simulink model "SF050A_MotTqTranlDampg"  (R2013b)
settings: Solver=FixedStepDiscrete  SolverMode=SingleTasking  StartTime=0.0  StopTime=29  FixedStep=.002  RelTol=1e-3
undefined symbols (not defined in the file): LoaSt1, MotTqTranlDampgCmdLim, MotTqTranlDampgDampgCoeff, MotTqTranlDampgRampEnd, MotTqTranlDampgTmrPt1, MotTqTranlDampgTmrPt2, MotTqTranlDampgVelThd, RAMPSTRT_ULS_U2P14, SYSGLBPRM_MOTTQCMDHILIM_MOTNWTMTR_F32, SYSGLBPRM_MOTTQCMDLOLIM_MOTNWTMTR_F32, SysSt1, TICNVN_MILLISECPERCNT_F32
libraries: simulink x8, FloatToFixd x4, FixdToFloat x3, NxtrSign x2, NxtrAbslt x1, LnrIntrpnDyn x1, LnrIntrpn x1
Description:
  | This FDD describes the controlled disable damping shutdown method used in the
  | EPS system for torque sensor failures.  When the torque sensor fails, an output
  | torque is computed based on motor velocity to reduce the amount of “handwheel
  | kick” perceived by the driver.
settings Model: Creator=Kevin Derry  LastModifiedBy=XZB1DB
settings OptimizationCC: ExpressionDepthLimit=2147483647

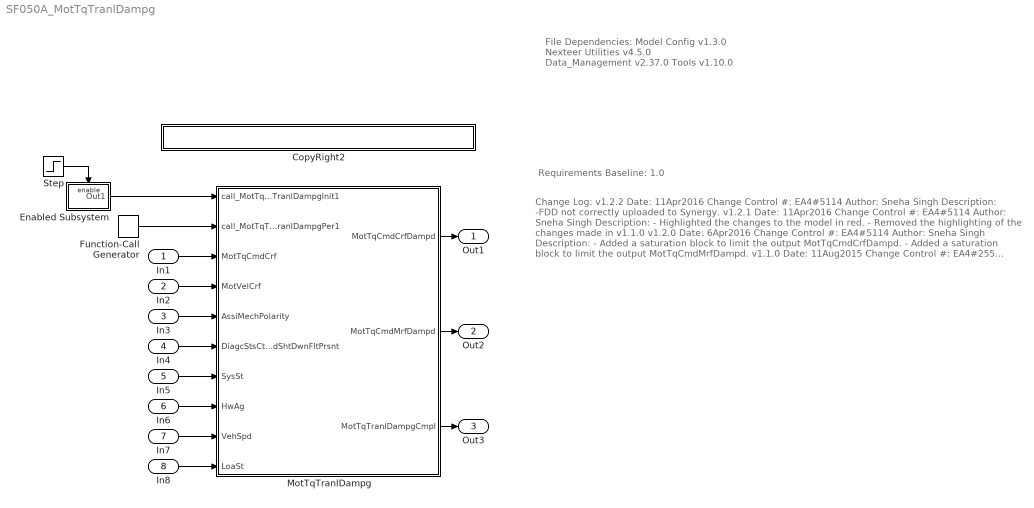
== system SF050A_MotTqTranlDampg ==
  note: File Dependencies:
      |
      | Model Config v1.3.0
      | Nexteer Utilities v4.5.0
      | Data_Management v2.37.0
      | Tools v1.10.0
  note: Requirements Baseline: 1.0
  note: Change Log:
      |
      | v1.2.2
      | Date: 11Apr2016
      | Change Control #: EA4#5114
      | Author: Sneha Singh
      | Description:
      | -FDD not correctly uploaded to Synergy.
      |
      | v1.2.1
      | Date: 11Apr2016
      | Change Control #: EA4#5114
      | Author: Sneha Singh
      | Description:
      | - Highlighted the changes to the model in red.
      | - Removed the highlighting of the changes made in v1.1.0
      |
      | v1.2.0
      | Date: 6Apr2016
      | Change Control #: EA4#5114
      | Author: Sneha Singh
      | Description:
      | - Added a saturation block to limit the output MotTqCmdCrfDampd.
      | - Added a saturation block to limit the output MotTqCmdMrfDampd.
      |
      | v1.1.0
      | Date:  11Aug2015
      | Change Control #: EA4#255
      | Author:  Kevin Derry
      | Description:
      | -  Datatype of CtrldDampgScaY was u16p0, now u2p14.
      | -  New RAMPSTRT constant used instead of hardcoded "1".
      | -  FixdToFloat after CtrldDampgSca interpolation was u16p0, now u2p14.
      | -  Verbiage of Reset Timer block reworded for clarity.
      | -  SwOutputCntrl block rearranged for clarity.  No functional change.
      | -  Datatype of cal MotTqTranlDampgRampEnd was f32, now u2p14.
      | -  Removed two FloatToFixd in MotTqTranlDampgInit1 runnable.
      |
      | v1.0.0
      | Date: 18July2015
      | Change Control #: EA4#255
      | Author:  Kevin Derry
      | Description:
      | - Initial Release, based on EA3 v002
      | - This is a "level zero" model, not fully compliant with
      |   EA4 standards (or even close to it, for that matter).
  In1 : Inport
  In2 : Inport  Port=2
  In3 : Inport  Port=3
  In4 : Inport  Port=4
  In5 : Inport  Port=5  OutDataTypeStr=Enum: SysSt1
  In6 : Inport  Port=6
  In7 : Inport  Port=7
  In8 : Inport  Port=8
  CopyRight2 : Subsystem  Description=|  mask(Copyright Information){none=on}
      | Copyright info block.                                               
      |                                                                     
      | Place copyright information at the top of every subsystem in design.
      mask prompts: none "No parameters"
      mask help: Place copyright information at the top of every subsystem in design.
      mask Display:
      | NxtrConf = 'Nexteer Confidential';
      | 
      | sys = bdroot; %handle for the current model ("system")
      | first = get_param(sys,'Created');
      | if(isempty(first))
      |     first = datestr(now,'yyyy');
      | else
      |     first = first(end-3:end);  %year is last four digits
      | end
      | 
      | last = get_param(sys,'LastModifiedDate');
      | if isempty(last)
      |     last = datestr(now,'yyyy');
      | else
      |     last = last(end-3:end);
      | end
      | 
      | if strcmp(first,last)
      |     fprintf('%s -- Copyright %s Nexteer',NxtrConf,first)
      | else
      |     fprintf('%s -- %s%s- %s Nexteer',NxtrConf,char(169),first,last)
      | end
  Enabled Subsystem : Subsystem  TreatAsAtomicUnit=on
  Function-Call Generator : simulink/Ports & Subsystems/Function-Call Generator  sample_time=.002  numberOfIterations=1
  MotTqTranlDampg : Subsystem
  Step : Step  Time=.0000001  Before=1  After=0  SampleTime=0
  Out1 : Outport
  Out2 : Outport  Port=2
  Out3 : Outport  Port=3
  wires:
  In8/1 -> MotTqTranlDampg/10(LoaSt)
  MotTqTranlDampg/1(MotTqCmdCrfDampd) -> Out1/1
  In5/1 -> MotTqTranlDampg/7(SysSt)
  In4/1 -> MotTqTranlDampg/6(DiagcStsCtrldShtDwnFltPrsnt)
  In6/1 -> MotTqTranlDampg/8(HwAg)
  In3/1 -> MotTqTranlDampg/5(AssiMechPolarity)
  In7/1 -> MotTqTranlDampg/9(VehSpd)
  In2/1 -> MotTqTranlDampg/4(MotVelCrf)
  In1/1 -> MotTqTranlDampg/3(MotTqCmdCrf)
  MotTqTranlDampg/2(MotTqCmdMrfDampd) -> Out2/1
  MotTqTranlDampg/3(MotTqTranlDampgCmpl) -> Out3/1
  Function-Call Generator/1 -> MotTqTranlDampg/2(call_MotTqTranlDampgPer1)
  Step/1 -> Enabled Subsystem/Enable
  Enabled Subsystem/1(Out1) -> MotTqTranlDampg/1(call_MotTqTranlDampgInit1)

== system SF050A_MotTqTranlDampg/CopyRight2 ==

== system SF050A_MotTqTranlDampg/Enabled Subsystem ==
  Enable : EnablePort
  Function-Call Generator1 : simulink/Ports & Subsystems/Function-Call Generator  sample_time=.002  numberOfIterations=1
  Out1 : Outport
  wires:
  Function-Call Generator1/1 -> Out1/1

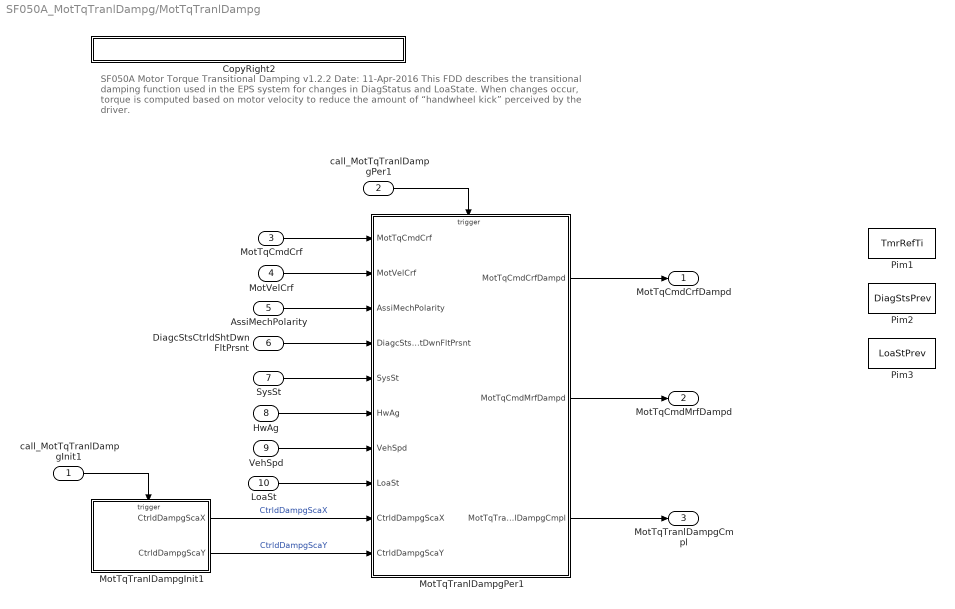
== system SF050A_MotTqTranlDampg/MotTqTranlDampg ==
  note: SF050A  Motor Torque Transitional Damping
      | v1.2.2      Date: 11-Apr-2016
      |
      | This FDD describes the transitional damping function used in the EPS system for changes in DiagStatus and LoaState.  When changes occur,
      | torque is computed based on motor velocity to reduce the amount of “handwheel kick” perceived by the driver.
  call_MotTqTranlDampgInit1 : Inport
  call_MotTqTranlDampgPer1 : Inport  Port=2
  MotTqCmdCrf : Inport  Port=3
  MotVelCrf : Inport  Port=4
  AssiMechPolarity : Inport  Port=5
  DiagcStsCtrldShtDwnFltPrsnt : Inport  Port=6
  SysSt : Inport  Port=7
  HwAg : Inport  Port=8
  VehSpd : Inport  Port=9
  LoaSt : Inport  Port=10
  CopyRight2 : Subsystem  Description=|  mask(Copyright Information){none=on}
      | Copyright info block.                                               
      |                                                                     
      | Place copyright information at the top of every subsystem in design.
      mask prompts: none "No parameters"
      mask help: Place copyright information at the top of every subsystem in design.
      mask Display:
      | NxtrConf = 'Nexteer Confidential';
      | 
      | sys = bdroot; %handle for the current model ("system")
      | first = get_param(sys,'Created');
      | if(isempty(first))
      |     first = datestr(now,'yyyy');
      | else
      |     first = first(end-3:end);  %year is last four digits
      | end
      | 
      | last = get_param(sys,'LastModifiedDate');
      | if isempty(last)
      |     last = datestr(now,'yyyy');
      | else
      |     last = last(end-3:end);
      | end
      | 
      | if strcmp(first,last)
      |     fprintf('%s -- Copyright %s Nexteer',NxtrConf,first)
      | else
      |     fprintf('%s -- %s%s- %s Nexteer',NxtrConf,char(169),first,last)
      | end
  MotTqTranlDampgInit1 : Subsystem
  MotTqTranlDampgPer1 : Subsystem
  Pim1 : DataStoreMemory  DataStoreName=TmrRefTi  ReadBeforeWriteMsg=warning  WriteAfterWriteMsg=warning  WriteAfterReadMsg=warning  StateMustResolveToSignalObject=on
  Pim2 : DataStoreMemory  DataStoreName=DiagStsPrev  ReadBeforeWriteMsg=warning  WriteAfterWriteMsg=warning  WriteAfterReadMsg=warning  StateMustResolveToSignalObject=on
  Pim3 : DataStoreMemory  DataStoreName=LoaStPrev  ReadBeforeWriteMsg=warning  WriteAfterWriteMsg=warning  WriteAfterReadMsg=warning  InitialValue=LoaSt1.LOAST_NORM  OutDataTypeStr=Enum: LoaSt1  StateMustResolveToSignalObject=on
  MotTqCmdCrfDampd : Outport
  MotTqCmdMrfDampd : Outport  Port=2
  MotTqTranlDampgCmpl : Outport  Port=3
  wires:
  MotTqCmdCrf/1 -> MotTqTranlDampgPer1/1(MotTqCmdCrf)
  MotVelCrf/1 -> MotTqTranlDampgPer1/2(MotVelCrf)
  AssiMechPolarity/1 -> MotTqTranlDampgPer1/3(AssiMechPolarity)
  DiagcStsCtrldShtDwnFltPrsnt/1 -> MotTqTranlDampgPer1/4(DiagcStsCtrldShtDwnFltPrsnt)
  SysSt/1 -> MotTqTranlDampgPer1/5(SysSt)
  HwAg/1 -> MotTqTranlDampgPer1/6(HwAg)
  VehSpd/1 -> MotTqTranlDampgPer1/7(VehSpd)
  LoaSt/1 -> MotTqTranlDampgPer1/8(LoaSt)
  MotTqTranlDampgPer1/1(MotTqCmdCrfDampd) -> MotTqCmdCrfDampd/1
  MotTqTranlDampgPer1/2(MotTqCmdMrfDampd) -> MotTqCmdMrfDampd/1
  MotTqTranlDampgPer1/3(MotTqTranlDampgCmpl) -> MotTqTranlDampgCmpl/1
  MotTqTranlDampgInit1/1(CtrldDampgScaX) -> MotTqTranlDampgPer1/9(CtrldDampgScaX)  "CtrldDampgScaX"
  MotTqTranlDampgInit1/2(CtrldDampgScaY) -> MotTqTranlDampgPer1/10(CtrldDampgScaY)  "CtrldDampgScaY"
  call_MotTqTranlDampgInit1/1 -> MotTqTranlDampgInit1/Trigger
  call_MotTqTranlDampgPer1/1 -> MotTqTranlDampgPer1/Trigger

== system SF050A_MotTqTranlDampg/MotTqTranlDampg/CopyRight2 ==

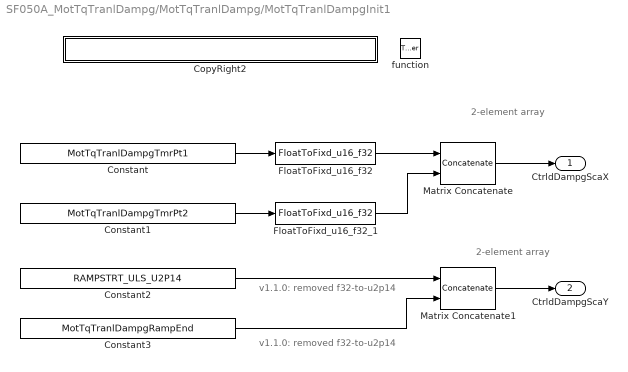
== system SF050A_MotTqTranlDampg/MotTqTranlDampg/MotTqTranlDampgInit1 ==
  note: v1.1.0: removed f32-to-u2p14
  note: 2-element array
  note: 2-element array
  note: v1.1.0: removed f32-to-u2p14
  function : TriggerPort  TriggerType=function-call
  Constant : Constant  Value=MotTqTranlDampgTmrPt1
  Constant1 : Constant  Value=MotTqTranlDampgTmrPt2
  Constant2 : Constant  Value=RAMPSTRT_ULS_U2P14
  Constant3 : Constant  Value=MotTqTranlDampgRampEnd
  CopyRight2 : Subsystem  Description=|  mask(Copyright Information){none=on}
      | Copyright info block.                                               
      |                                                                     
      | Place copyright information at the top of every subsystem in design.
      mask prompts: none "No parameters"
      mask help: Place copyright information at the top of every subsystem in design.
      mask Display:
      | NxtrConf = 'Nexteer Confidential';
      | 
      | sys = bdroot; %handle for the current model ("system")
      | first = get_param(sys,'Created');
      | if(isempty(first))
      |     first = datestr(now,'yyyy');
      | else
      |     first = first(end-3:end);  %year is last four digits
      | end
      | 
      | last = get_param(sys,'LastModifiedDate');
      | if isempty(last)
      |     last = datestr(now,'yyyy');
      | else
      |     last = last(end-3:end);
      | end
      | 
      | if strcmp(first,last)
      |     fprintf('%s -- Copyright %s Nexteer',NxtrConf,first)
      | else
      |     fprintf('%s -- %s%s- %s Nexteer',NxtrConf,char(169),first,last)
      | end
  FloatToFixd_u16_f32 : FloatToFixd/FloatToFixd_u16_f32  Param1=0
  FloatToFixd_u16_f32_1 : FloatToFixd/FloatToFixd_u16_f32  Param1=0
  Matrix Concatenate : Concatenate
  Matrix Concatenate1 : Concatenate
  CtrldDampgScaX : Outport
  CtrldDampgScaY : Outport  Port=2
  wires:
  Constant/1 -> FloatToFixd_u16_f32/1
  Constant1/1 -> FloatToFixd_u16_f32_1/1
  FloatToFixd_u16_f32/1 -> Matrix Concatenate/1
  FloatToFixd_u16_f32_1/1 -> Matrix Concatenate/2
  Constant2/1 -> Matrix Concatenate1/1
  Constant3/1 -> Matrix Concatenate1/2
  Matrix Concatenate1/1 -> CtrldDampgScaY/1
  Matrix Concatenate/1 -> CtrldDampgScaX/1

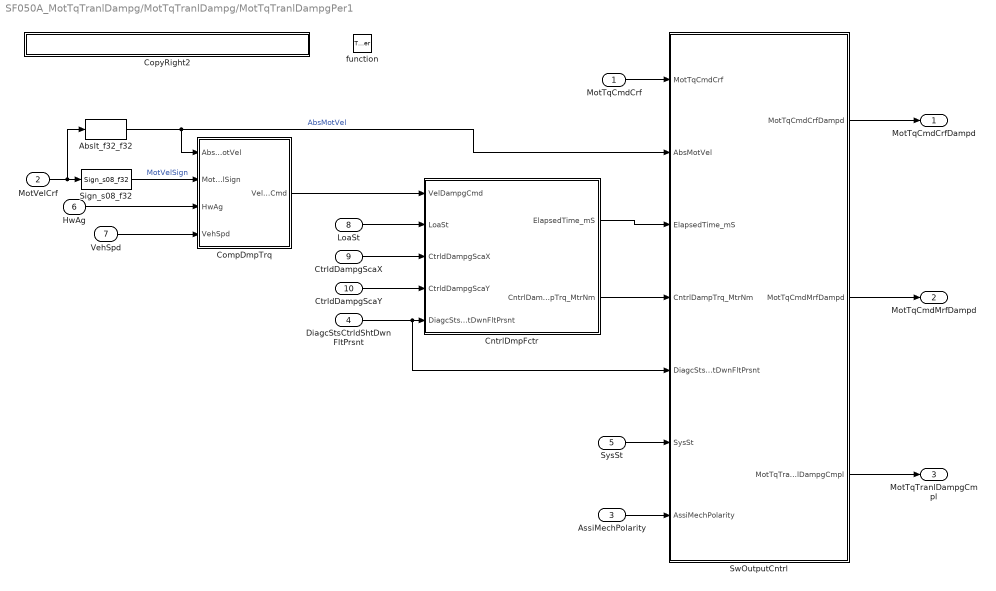
== system SF050A_MotTqTranlDampg/MotTqTranlDampg/MotTqTranlDampgPer1 ==
  MotTqCmdCrf : Inport
  MotVelCrf : Inport  Port=2
  AssiMechPolarity : Inport  Port=3
  DiagcStsCtrldShtDwnFltPrsnt : Inport  Port=4
  SysSt : Inport  Port=5
  HwAg : Inport  Port=6
  VehSpd : Inport  Port=7
  LoaSt : Inport  Port=8
  CtrldDampgScaX : Inport  Port=9
  CtrldDampgScaY : Inport  Port=10
  function : TriggerPort  TriggerType=function-call
  Abslt_f32_f32 : NxtrAbslt/Abslt_f32_f32  SFunctionSpec=single y1 = Abslt_f32_f32(single u1)
      settings: AttributesFormatString=%<Name>
  CntrlDmpFctr : Subsystem  Tag=Control Damping Factor
      settings: AttributesFormatString=%<Tag>
  CompDmpTrq : Subsystem  Tag=Compute Damping Torque
      settings: AttributesFormatString=%<Tag>
  CopyRight2 : Subsystem  Description=|  mask(Copyright Information){none=on}
      | Copyright info block.                                               
      |                                                                     
      | Place copyright information at the top of every subsystem in design.
      mask prompts: none "No parameters"
      mask help: Place copyright information at the top of every subsystem in design.
      mask Display:
      | NxtrConf = 'Nexteer Confidential';
      | 
      | sys = bdroot; %handle for the current model ("system")
      | first = get_param(sys,'Created');
      | if(isempty(first))
      |     first = datestr(now,'yyyy');
      | else
      |     first = first(end-3:end);  %year is last four digits
      | end
      | 
      | last = get_param(sys,'LastModifiedDate');
      | if isempty(last)
      |     last = datestr(now,'yyyy');
      | else
      |     last = last(end-3:end);
      | end
      | 
      | if strcmp(first,last)
      |     fprintf('%s -- Copyright %s Nexteer',NxtrConf,first)
      | else
      |     fprintf('%s -- %s%s- %s Nexteer',NxtrConf,char(169),first,last)
      | end
  Sign_s08_f32 : NxtrSign/Sign_s08_f32  SFunctionSpec=int8 y1 = Sign_s08_f32(single u1)
  SwOutputCntrl : Subsystem  Tag=Switch Output Control
      settings: AttributesFormatString=%<Tag>
  MotTqCmdCrfDampd : Outport
  MotTqCmdMrfDampd : Outport  Port=2
  MotTqTranlDampgCmpl : Outport  Port=3
  wires:
  DiagcStsCtrldShtDwnFltPrsnt/1 -> SwOutputCntrl/5(DiagcStsCtrldShtDwnFltPrsnt), CntrlDmpFctr/5(DiagcStsCtrldShtDwnFltPrsnt)
  LoaSt/1 -> CntrlDmpFctr/2(LoaSt)
  SysSt/1 -> SwOutputCntrl/6(SysSt)
  CntrlDmpFctr/2(CntrlDampTrq_MtrNm) -> SwOutputCntrl/4(CntrlDampTrq_MtrNm)
  CompDmpTrq/1(VelDampgCmd) -> CntrlDmpFctr/1(VelDampgCmd)
  MotTqCmdCrf/1 -> SwOutputCntrl/1(MotTqCmdCrf)
  SwOutputCntrl/1(MotTqCmdCrfDampd) -> MotTqCmdCrfDampd/1
  SwOutputCntrl/2(MotTqCmdMrfDampd) -> MotTqCmdMrfDampd/1
  SwOutputCntrl/3(MotTqTranlDampgCmpl) -> MotTqTranlDampgCmpl/1
  CntrlDmpFctr/1(ElapsedTime_mS) -> SwOutputCntrl/3(ElapsedTime_mS)
  AssiMechPolarity/1 -> SwOutputCntrl/7(AssiMechPolarity)
  CtrldDampgScaX/1 -> CntrlDmpFctr/3(CtrldDampgScaX)
  CtrldDampgScaY/1 -> CntrlDmpFctr/4(CtrldDampgScaY)
  MotVelCrf/1 -> Abslt_f32_f32/1, Sign_s08_f32/1
  Sign_s08_f32/1 -> CompDmpTrq/2(MotVelSign)  "MotVelSign"
  Abslt_f32_f32/1 -> CompDmpTrq/1(AbsMotVel), SwOutputCntrl/2(AbsMotVel)  "AbsMotVel"
  HwAg/1 -> CompDmpTrq/3(HwAg)
  VehSpd/1 -> CompDmpTrq/4(VehSpd)

== system SF050A_MotTqTranlDampg/MotTqTranlDampg/MotTqTranlDampgInit1/CopyRight2 ==

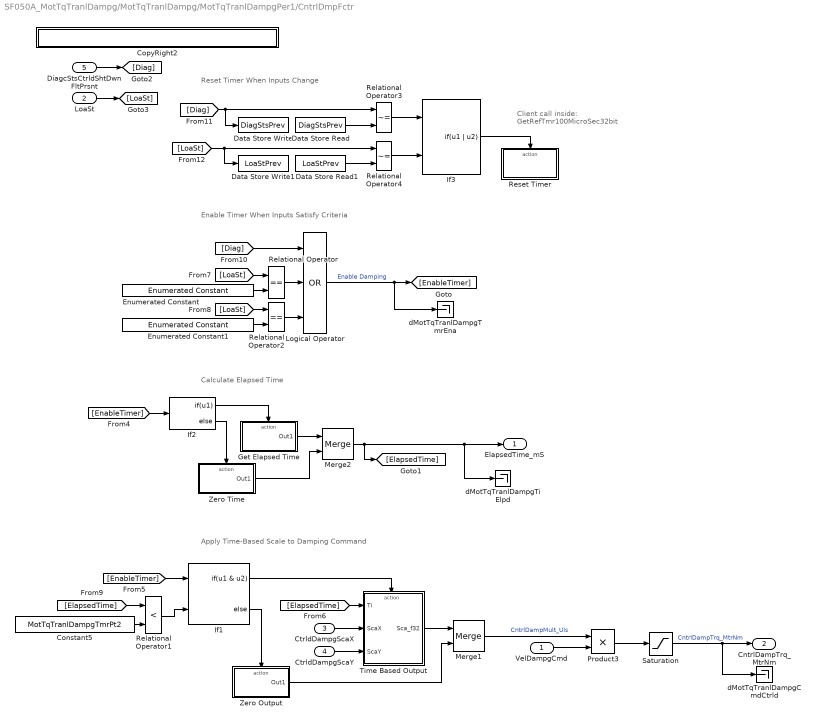
== system SF050A_MotTqTranlDampg/MotTqTranlDampg/MotTqTranlDampgPer1/CntrlDmpFctr ==
  note: Reset Timer When Inputs Change
  note: Client call inside:
      | GetRefTmr100MicroSec32bit
  note: Enable Timer When Inputs Satisfy Criteria
  note: Calculate Elapsed Time
  note: Apply Time-Based Scale to Damping Command
  VelDampgCmd : Inport
  LoaSt : Inport  Port=2
  CtrldDampgScaX : Inport  Port=3
  CtrldDampgScaY : Inport  Port=4
  DiagcStsCtrldShtDwnFltPrsnt : Inport  Port=5
  Constant5 : Constant  Value=MotTqTranlDampgTmrPt2
  CopyRight2 : Subsystem  Description=|  mask(Copyright Information){none=on}
      | Copyright info block.                                               
      |                                                                     
      | Place copyright information at the top of every subsystem in design.
      mask prompts: none "No parameters"
      mask help: Place copyright information at the top of every subsystem in design.
      mask Display:
      | NxtrConf = 'Nexteer Confidential';
      | 
      | sys = bdroot; %handle for the current model ("system")
      | first = get_param(sys,'Created');
      | if(isempty(first))
      |     first = datestr(now,'yyyy');
      | else
      |     first = first(end-3:end);  %year is last four digits
      | end
      | 
      | last = get_param(sys,'LastModifiedDate');
      | if isempty(last)
      |     last = datestr(now,'yyyy');
      | else
      |     last = last(end-3:end);
      | end
      | 
      | if strcmp(first,last)
      |     fprintf('%s -- Copyright %s Nexteer',NxtrConf,first)
      | else
      |     fprintf('%s -- %s%s- %s Nexteer',NxtrConf,char(169),first,last)
      | end
  Data Store Read : DataStoreRead  Priority=1  DataStoreName=DiagStsPrev
  Data Store Read1 : DataStoreRead  Priority=1  DataStoreName=LoaStPrev
  Data Store Write : DataStoreWrite  Priority=2  DataStoreName=DiagStsPrev
  Data Store Write1 : DataStoreWrite  Priority=2  DataStoreName=LoaStPrev
  Enumerated Constant : simulink/Sources/Enumerated Constant  OutDataTypeStr=Enum: LoaSt1  Value=LoaSt1.LOAST_SWBASDMTGTN  SampleTime=inf
  Enumerated Constant1 : simulink/Sources/Enumerated Constant  OutDataTypeStr=Enum: LoaSt1  Value=LoaSt1.LOAST_FADEOUT  SampleTime=inf
  Get Elapsed Time : Subsystem  TreatAsAtomicUnit=on
  If1 : If  NumInputs=2  IfExpression=u1 & u2
  If2 : If  IfExpression=u1
  If3 : If  NumInputs=2  IfExpression=u1 | u2  ShowElse=off
  Logical Operator : Logic  Operator=OR  Inputs=3  AllPortsSameDT=off  OutDataTypeStr=boolean
  Merge1 : Merge
  Merge2 : Merge
  Product3 : Product  RndMeth=Zero
  Relational Operator : RelationalOperator  Operator===  OutDataTypeStr=boolean
  Relational Operator1 : RelationalOperator  Operator=<  OutDataTypeStr=boolean
  Relational Operator2 : RelationalOperator  Operator===  OutDataTypeStr=boolean
  Relational Operator3 : RelationalOperator  Operator=~=  OutDataTypeStr=boolean
  Relational Operator4 : RelationalOperator  Operator=~=  OutDataTypeStr=boolean
  Reset Timer : Subsystem  TreatAsAtomicUnit=on
  Saturation : Saturate  UpperLimit=MotTqTranlDampgCmdLim  LowerLimit=-MotTqTranlDampgCmdLim
      settings: AttributesFormatString=%<UpperLimit>\n%<LowerLimit>
  Time Based Output : Subsystem  TreatAsAtomicUnit=on
  Zero Output : Subsystem  TreatAsAtomicUnit=on
  Zero Time : Subsystem  TreatAsAtomicUnit=on
  dMotTqTranlDampgCmdCtrld : Terminator
  "dMotTqTranlDampgTiElpd   " : Terminator
  "dMotTqTranlDampgTmrEna   " : Terminator
  ElapsedTime_mS : Outport
  CntrlDampTrq_MtrNm : Outport  Port=2
  wires:
  Saturation/1 -> dMotTqTranlDampgCmdCtrld/1, CntrlDampTrq_MtrNm/1  "CntrlDampTrq_MtrNm"
  Constant5/1 -> Relational Operator1/2
  Merge1/1 -> Product3/1  "CntrlDampMult_Uls"
  VelDampgCmd/1 -> Product3/2
  Product3/1 -> Saturation/1
  DiagcStsCtrldShtDwnFltPrsnt/1 -> [Diag]
  Merge2/1 -> ElapsedTime_mS/1, "dMotTqTranlDampgTiElpd   "/1, [ElapsedTime]
  [ElapsedTime] -> Relational Operator1/1
  Relational Operator1/1 -> If1/2
  Enumerated Constant/1 -> Relational Operator/2
  Enumerated Constant1/1 -> Relational Operator2/2
  [ElapsedTime] -> Time Based Output/1(Ti)
  CtrldDampgScaX/1 -> Time Based Output/2(ScaX)
  CtrldDampgScaY/1 -> Time Based Output/3(ScaY)
  If1/1 -> Time Based Output/Action
  [EnableTimer] -> If1/1
  If1/2 -> Zero Output/Action
  Time Based Output/1(Sca_f32) -> Merge1/1
  Zero Output/1(Out1) -> Merge1/2
  [EnableTimer] -> If2/1
  If2/2 -> Zero Time/Action
  If2/1 -> Get Elapsed Time/Action
  Get Elapsed Time/1(Out1) -> Merge2/1
  Zero Time/1(Out1) -> Merge2/2
  Logical Operator/1 -> [EnableTimer], "dMotTqTranlDampgTmrEna   "/1  "Enable Damping"
  LoaSt/1 -> [LoaSt]
  [LoaSt] -> Relational Operator/1
  [LoaSt] -> Relational Operator2/1
  Relational Operator/1 -> Logical Operator/2
  Relational Operator2/1 -> Logical Operator/3
  [Diag] -> Logical Operator/1
  [Diag] -> Data Store Write/1, Relational Operator3/1
  Data Store Read1/1 -> Relational Operator4/2
  [LoaSt] -> Data Store Write1/1, Relational Operator4/1
  Relational Operator3/1 -> If3/1
  Relational Operator4/1 -> If3/2
  If3/1 -> Reset Timer/Action
  Data Store Read/1 -> Relational Operator3/2

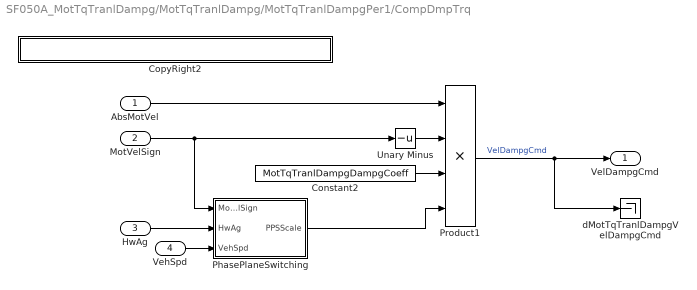
== system SF050A_MotTqTranlDampg/MotTqTranlDampg/MotTqTranlDampgPer1/CompDmpTrq ==
  AbsMotVel : Inport
  MotVelSign : Inport  Port=2
  HwAg : Inport  Port=3
  VehSpd : Inport  Port=4
  Constant2 : Constant  Value=MotTqTranlDampgDampgCoeff
  CopyRight2 : Subsystem  Description=|  mask(Copyright Information){none=on}
      | Copyright info block.                                               
      |                                                                     
      | Place copyright information at the top of every subsystem in design.
      mask prompts: none "No parameters"
      mask help: Place copyright information at the top of every subsystem in design.
      mask Display:
      | NxtrConf = 'Nexteer Confidential';
      | 
      | sys = bdroot; %handle for the current model ("system")
      | first = get_param(sys,'Created');
      | if(isempty(first))
      |     first = datestr(now,'yyyy');
      | else
      |     first = first(end-3:end);  %year is last four digits
      | end
      | 
      | last = get_param(sys,'LastModifiedDate');
      | if isempty(last)
      |     last = datestr(now,'yyyy');
      | else
      |     last = last(end-3:end);
      | end
      | 
      | if strcmp(first,last)
      |     fprintf('%s -- Copyright %s Nexteer',NxtrConf,first)
      | else
      |     fprintf('%s -- %s%s- %s Nexteer',NxtrConf,char(169),first,last)
      | end
  PhasePlaneSwitching : Subsystem
  Product1 : Product  Inputs=4  OutDataTypeStr=single  RndMeth=Zero
  Unary Minus : UnaryMinus
  "dMotTqTranlDampgVelDampgCmd " : Terminator
  VelDampgCmd : Outport
  wires:
  MotVelSign/1 -> Unary Minus/1, PhasePlaneSwitching/1(MotVelSign)
  Unary Minus/1 -> Product1/2
  Product1/1 -> "dMotTqTranlDampgVelDampgCmd "/1, VelDampgCmd/1  "VelDampgCmd"
  Constant2/1 -> Product1/3
  HwAg/1 -> PhasePlaneSwitching/2(HwAg)
  VehSpd/1 -> PhasePlaneSwitching/3(VehSpd)
  PhasePlaneSwitching/1(PPSScale) -> Product1/4
  AbsMotVel/1 -> Product1/1

== system SF050A_MotTqTranlDampg/MotTqTranlDampg/MotTqTranlDampgPer1/CopyRight2 ==

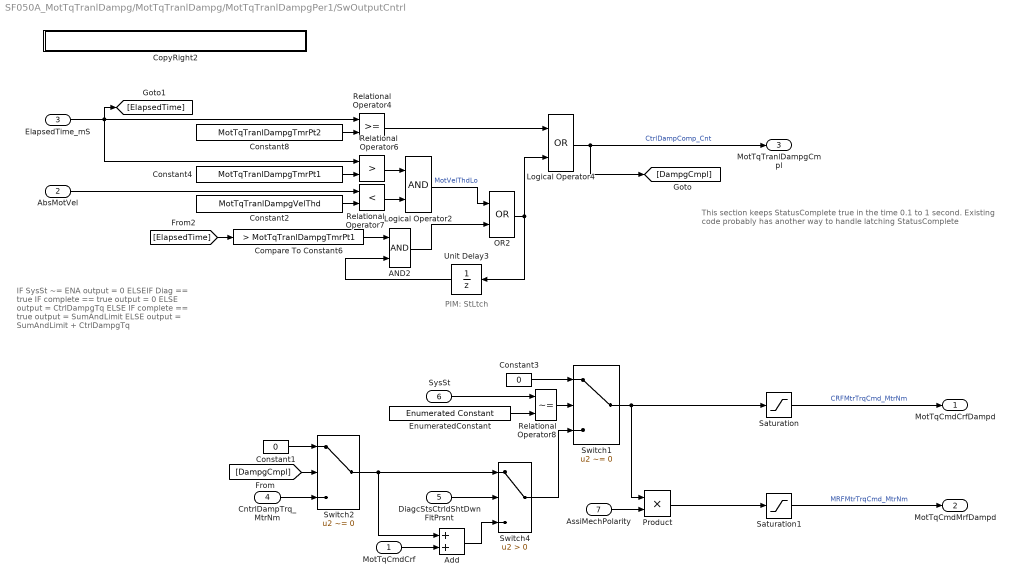
== system SF050A_MotTqTranlDampg/MotTqTranlDampg/MotTqTranlDampgPer1/SwOutputCntrl ==
  note: PIM: StLtch
  note: IF  SysSt ~= ENA
      |    output = 0
      | ELSEIF  Diag == true
      |    IF  complete == true
      |        output = 0
      |    ELSE
      |        output = CtrlDampgTq
      | ELSE
      |    IF  complete == true
      |        output = SumAndLimit
      |    ELSE
      |        output = SumAndLimit + CtrlDampgTq
  note: This section keeps StatusComplete true in the time 0.1 to 1 second.
      | Existing code probably has another way to handle latching StatusComplete
  MotTqCmdCrf : Inport
  AbsMotVel : Inport  Port=2
  ElapsedTime_mS : Inport  Port=3
  CntrlDampTrq_MtrNm : Inport  Port=4
  DiagcStsCtrldShtDwnFltPrsnt : Inport  Port=5
  SysSt : Inport  Port=6
  AssiMechPolarity : Inport  Port=7
  AND2 : Logic  AllPortsSameDT=off
  Add : Sum
  Compare To Constant6 : simulink/Logic and Bit Operations/Compare To Constant  relop=>  const=MotTqTranlDampgTmrPt1  OutDataTypeStr=boolean
  Constant1 : Constant  Value=0  OutDataTypeStr=single
  Constant2 : Constant  Value=MotTqTranlDampgVelThd
  Constant3 : Constant  Value=0  OutDataTypeStr=single
  Constant4 : Constant  Value=MotTqTranlDampgTmrPt1
  Constant8 : Constant  Value=MotTqTranlDampgTmrPt2
  CopyRight2 : Subsystem  Description=|  mask(Copyright Information){none=on}
      | Copyright info block.                                               
      |                                                                     
      | Place copyright information at the top of every subsystem in design.
      mask prompts: none "No parameters"
      mask help: Place copyright information at the top of every subsystem in design.
      mask Display:
      | NxtrConf = 'Nexteer Confidential';
      | 
      | sys = bdroot; %handle for the current model ("system")
      | first = get_param(sys,'Created');
      | if(isempty(first))
      |     first = datestr(now,'yyyy');
      | else
      |     first = first(end-3:end);  %year is last four digits
      | end
      | 
      | last = get_param(sys,'LastModifiedDate');
      | if isempty(last)
      |     last = datestr(now,'yyyy');
      | else
      |     last = last(end-3:end);
      | end
      | 
      | if strcmp(first,last)
      |     fprintf('%s -- Copyright %s Nexteer',NxtrConf,first)
      | else
      |     fprintf('%s -- %s%s- %s Nexteer',NxtrConf,char(169),first,last)
      | end
  EnumeratedConstant : simulink/Sources/Enumerated Constant  OutDataTypeStr=Enum: SysSt1  Value=SysSt1.SYSST_ENA  SampleTime=inf
  Logical Operator2 : Logic  AllPortsSameDT=off  OutDataTypeStr=boolean
  Logical Operator4 : Logic  Operator=OR  AllPortsSameDT=off  OutDataTypeStr=boolean
  OR2 : Logic  Operator=OR  AllPortsSameDT=off  OutDataTypeStr=boolean
  Product : Product  RndMeth=Zero
  Relational Operator4 : RelationalOperator  OutDataTypeStr=boolean
  Relational Operator6 : RelationalOperator  Operator=>  OutDataTypeStr=boolean
  Relational Operator7 : RelationalOperator  Operator=<  OutDataTypeStr=boolean
  Relational Operator8 : RelationalOperator  Operator=~=  OutDataTypeStr=boolean
  Saturation : Saturate  UpperLimit=SYSGLBPRM_MOTTQCMDHILIM_MOTNWTMTR_F32  LowerLimit=SYSGLBPRM_MOTTQCMDLOLIM_MOTNWTMTR_F32
      settings: AttributesFormatString=|
      | LowerLimit=%<LowerLimit>
      | UpperLimit=%<UpperLimit>
  Saturation1 : Saturate  UpperLimit=SYSGLBPRM_MOTTQCMDHILIM_MOTNWTMTR_F32  LowerLimit=SYSGLBPRM_MOTTQCMDLOLIM_MOTNWTMTR_F32
      settings: AttributesFormatString=|
      | LowerLimit=%<LowerLimit>
      | UpperLimit=%<UpperLimit>
  Switch1 : Switch  Criteria=u2 ~= 0  Threshold=1
  Switch2 : Switch  Criteria=u2 ~= 0  Threshold=1
  Switch4 : Switch  Criteria=u2 > Threshold
  Unit Delay3 : UnitDelay  SampleTime=-1  StateName=StLtch  StateMustResolveToSignalObject=on
  MotTqCmdCrfDampd : Outport
  MotTqCmdMrfDampd : Outport  Port=2
  MotTqTranlDampgCmpl : Outport  Port=3
  wires:
  Product/1 -> Saturation1/1
  Switch1/1 -> Saturation/1, Product/1
  CntrlDampTrq_MtrNm/1 -> Switch2/3
  MotTqCmdCrf/1 -> Add/2
  AbsMotVel/1 -> Relational Operator7/1
  Constant8/1 -> Relational Operator4/2
  Relational Operator7/1 -> Logical Operator2/2
  Relational Operator6/1 -> Logical Operator2/1
  Constant2/1 -> Relational Operator7/2
  Constant4/1 -> Relational Operator6/2
  Relational Operator4/1 -> Logical Operator4/1
  ElapsedTime_mS/1 -> Relational Operator4/1, [ElapsedTime], Relational Operator6/1
  Logical Operator4/1 -> MotTqTranlDampgCmpl/1, [DampgCmpl]  "CtrlDampComp_Cnt"
  SysSt/1 -> Relational Operator8/1
  EnumeratedConstant/1 -> Relational Operator8/2
  Relational Operator8/1 -> Switch1/2
  Constant3/1 -> Switch1/1
  Switch4/1 -> Switch1/3
  DiagcStsCtrldShtDwnFltPrsnt/1 -> Switch4/2
  Constant1/1 -> Switch2/1
  Switch2/1 -> Switch4/1, Add/1
  Add/1 -> Switch4/3
  [DampgCmpl] -> Switch2/2
  OR2/1 -> Logical Operator4/2, Unit Delay3/1
  [ElapsedTime] -> Compare To Constant6/1
  AND2/1 -> OR2/2
  Logical Operator2/1 -> OR2/1  "MotVelThdLo"
  AssiMechPolarity/1 -> Product/2
  Compare To Constant6/1 -> AND2/1
  Unit Delay3/1 -> AND2/2
  Saturation/1 -> MotTqCmdCrfDampd/1  "CRFMtrTrqCmd_MtrNm"
  Saturation1/1 -> MotTqCmdMrfDampd/1  "MRFMtrTrqCmd_MtrNm"

== system SF050A_MotTqTranlDampg/MotTqTranlDampg/MotTqTranlDampgPer1/CntrlDmpFctr/CopyRight2 ==

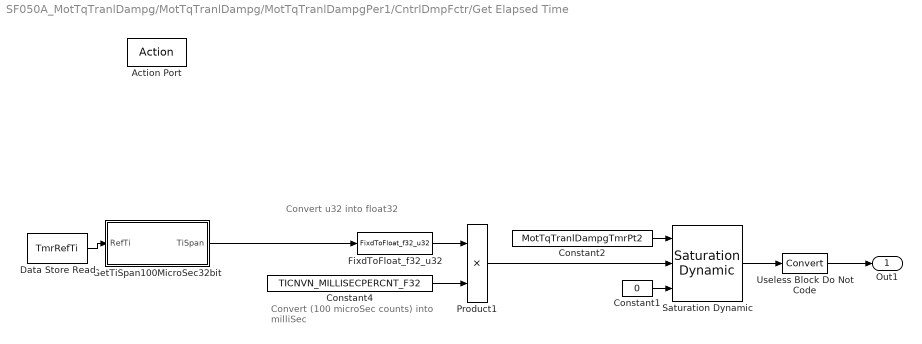
== system SF050A_MotTqTranlDampg/MotTqTranlDampg/MotTqTranlDampgPer1/CntrlDmpFctr/Get Elapsed Time ==
  note: Convert u32 into float32
  note: Convert (100 microSec counts)
      | into  milliSec
  Action Port : ActionPort  ActionType=then
  Constant1 : Constant  Value=0  OutDataTypeStr=single
  Constant2 : Constant  Value=MotTqTranlDampgTmrPt2
  Constant4 : Constant  Value=TICNVN_MILLISECPERCNT_F32
  Data Store Read : DataStoreRead  DataStoreName=TmrRefTi
  FixdToFloat_f32_u32 : FixdToFloat/FixdToFloat_f32_u32  Param1=0
  GetTiSpan100MicroSec32bit : Subsystem
  Product1 : Product  RndMeth=Zero
  Saturation Dynamic : simulink/Discontinuities/Saturation Dynamic  OutMin=[]  OutMax=[]  OutDataTypeStr=Inherit: Same as second input  OutDataType=fixdt(1, 16)  OutScaling=2^-10  DoSatur=off
  Useless Block Do Not Code : DataTypeConversion
  Out1 : Outport
  wires:
  Constant1/1 -> Saturation Dynamic/3
  Constant2/1 -> Saturation Dynamic/1
  Data Store Read/1 -> GetTiSpan100MicroSec32bit/1(RefTi)
  Constant4/1 -> Product1/2
  GetTiSpan100MicroSec32bit/1(TiSpan) -> FixdToFloat_f32_u32/1
  Product1/1 -> Saturation Dynamic/2
  Saturation Dynamic/1 -> Useless Block Do Not Code/1
  FixdToFloat_f32_u32/1 -> Product1/1
  Useless Block Do Not Code/1 -> Out1/1

== system SF050A_MotTqTranlDampg/MotTqTranlDampg/MotTqTranlDampgPer1/CntrlDmpFctr/Reset Timer ==
  note: Write the reference time to PIM so it can be used to
      | get elapsed time in this and subsequent execution loops.
  Action Port : ActionPort  ActionType=then
  Data Store Write : DataStoreWrite  DataStoreName=TmrRefTi
  GetRefTmr100MicroSec32bit : Subsystem
  wires:
  GetRefTmr100MicroSec32bit/1(RefTi) -> Data Store Write/1

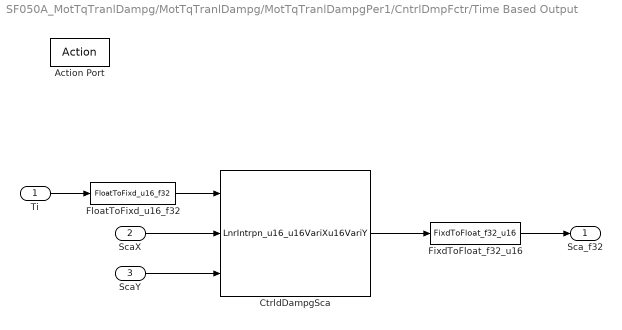
== system SF050A_MotTqTranlDampg/MotTqTranlDampg/MotTqTranlDampgPer1/CntrlDmpFctr/Time Based Output ==
  Ti : Inport
  ScaX : Inport  Port=2
  ScaY : Inport  Port=3
  Action Port : ActionPort  ActionType=then
  CtrldDampgSca : LnrIntrpnDyn/LnrIntrpn_u16_u16VariXu16VariY
      settings: AttributesFormatString=Lnr ( u16VariX , u16VariY )
  FixdToFloat_f32_u16 : FixdToFloat/FixdToFloat_f32_u16  Param1=14
  FloatToFixd_u16_f32 : FloatToFixd/FloatToFixd_u16_f32  Param1=0
  Sca_f32 : Outport
  wires:
  CtrldDampgSca/1 -> FixdToFloat_f32_u16/1
  Ti/1 -> FloatToFixd_u16_f32/1
  ScaX/1 -> CtrldDampgSca/2
  ScaY/1 -> CtrldDampgSca/3
  FixdToFloat_f32_u16/1 -> Sca_f32/1
  FloatToFixd_u16_f32/1 -> CtrldDampgSca/1

== system SF050A_MotTqTranlDampg/MotTqTranlDampg/MotTqTranlDampgPer1/CntrlDmpFctr/Zero Output ==
  Action Port : ActionPort  ActionType=else
  Constant : Constant  Value=0  OutDataTypeStr=single
  Out1 : Outport
  wires:
  Constant/1 -> Out1/1

== system SF050A_MotTqTranlDampg/MotTqTranlDampg/MotTqTranlDampgPer1/CntrlDmpFctr/Zero Time ==
  Action Port : ActionPort  ActionType=else
  Constant : Constant  Value=0  OutDataTypeStr=single
  Out1 : Outport
  wires:
  Constant/1 -> Out1/1

== system SF050A_MotTqTranlDampg/MotTqTranlDampg/MotTqTranlDampgPer1/CompDmpTrq/CopyRight2 ==

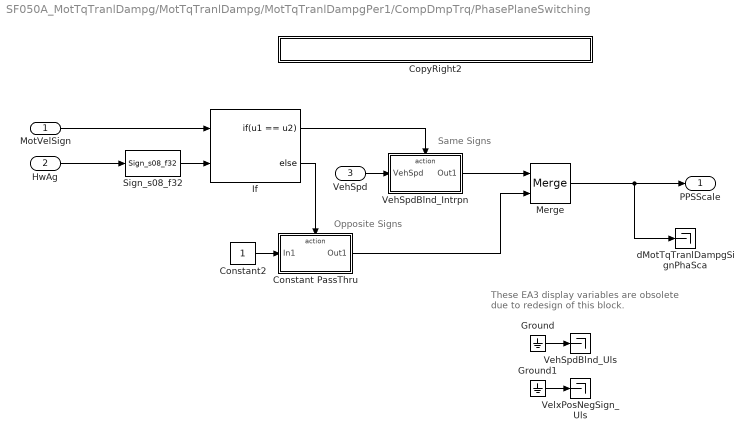
== system SF050A_MotTqTranlDampg/MotTqTranlDampg/MotTqTranlDampgPer1/CompDmpTrq/PhasePlaneSwitching ==
  note: These EA3 display variables are obsolete
      | due to redesign of this block.
  note: Opposite Signs
  note: Same Signs
  MotVelSign : Inport
  HwAg : Inport  Port=2
  VehSpd : Inport  Port=3
  Constant PassThru : Subsystem  TreatAsAtomicUnit=on
  Constant2 : Constant  OutDataTypeStr=single
  CopyRight2 : Subsystem  Description=|  mask(Copyright Information){none=on}
      | Copyright info block.                                               
      |                                                                     
      | Place copyright information at the top of every subsystem in design.
      mask prompts: none "No parameters"
      mask help: Place copyright information at the top of every subsystem in design.
      mask Display:
      | NxtrConf = 'Nexteer Confidential';
      | 
      | sys = bdroot; %handle for the current model ("system")
      | first = get_param(sys,'Created');
      | if(isempty(first))
      |     first = datestr(now,'yyyy');
      | else
      |     first = first(end-3:end);  %year is last four digits
      | end
      | 
      | last = get_param(sys,'LastModifiedDate');
      | if isempty(last)
      |     last = datestr(now,'yyyy');
      | else
      |     last = last(end-3:end);
      | end
      | 
      | if strcmp(first,last)
      |     fprintf('%s -- Copyright %s Nexteer',NxtrConf,first)
      | else
      |     fprintf('%s -- %s%s- %s Nexteer',NxtrConf,char(169),first,last)
      | end
  Ground : Ground
  Ground1 : Ground
  If : If  NumInputs=2  IfExpression=u1 == u2
  Merge : Merge
  Sign_s08_f32 : NxtrSign/Sign_s08_f32  SFunctionSpec=int8 y1 = Sign_s08_f32(single u1)
  VehSpdBlnd_Intrpn : Subsystem  TreatAsAtomicUnit=on
  VehSpdBlnd_Uls : Terminator
  VelxPosNegSign_Uls : Terminator
  "dMotTqTranlDampgSignPhaSca   " : Terminator
  PPSScale : Outport
  wires:
  MotVelSign/1 -> If/1
  Sign_s08_f32/1 -> If/2
  HwAg/1 -> Sign_s08_f32/1
  Constant2/1 -> Constant PassThru/1(In1)
  VehSpd/1 -> VehSpdBlnd_Intrpn/1(VehSpd)
  If/1 -> VehSpdBlnd_Intrpn/Action
  If/2 -> Constant PassThru/Action
  VehSpdBlnd_Intrpn/1(Out1) -> Merge/1
  Constant PassThru/1(Out1) -> Merge/2
  Merge/1 -> "dMotTqTranlDampgSignPhaSca   "/1, PPSScale/1
  Ground/1 -> VehSpdBlnd_Uls/1
  Ground1/1 -> VelxPosNegSign_Uls/1

== system SF050A_MotTqTranlDampg/MotTqTranlDampg/MotTqTranlDampgPer1/SwOutputCntrl/CopyRight2 ==

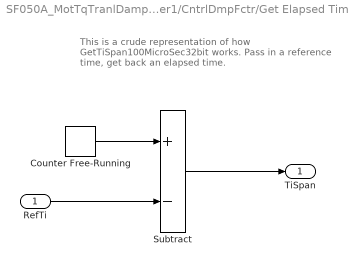
== system SF050A_MotTqTranlDampg/MotTqTranlDampg/MotTqTranlDampgPer1/CntrlDmpFctr/Get Elapsed Time/GetTiSpan100MicroSec32bit ==
  note: This is a crude representation of how
      | GetTiSpan100MicroSec32bit works.
      | Pass in a reference time, get back an
      | elapsed time.
  RefTi : Inport
  Counter Free-Running : simulink/Sources/Counter Free-Running  NumBits=32  tsamp=-1
  Subtract : Sum  Inputs=+-  OutDataTypeStr=uint32
  TiSpan : Outport
  wires:
  Counter Free-Running/1 -> Subtract/1
  RefTi/1 -> Subtract/2
  Subtract/1 -> TiSpan/1

== system SF050A_MotTqTranlDampg/MotTqTranlDampg/MotTqTranlDampgPer1/CntrlDmpFctr/Reset Timer/GetRefTmr100MicroSec32bit ==
  note: This represents a client call to GetRefTmr100MicroSec32bit.
      | This junky model always assumes the value returned is
      | a zero.  Code will behave differently.
  Constant : Constant  Value=0
  Data Type Conversion : DataTypeConversion  OutDataTypeStr=uint32
  RefTi : Outport
  wires:
  Constant/1 -> Data Type Conversion/1
  Data Type Conversion/1 -> RefTi/1

== system SF050A_MotTqTranlDampg/MotTqTranlDampg/MotTqTranlDampgPer1/CompDmpTrq/PhasePlaneSwitching/Constant PassThru ==
  In1 : Inport
  Action Port : ActionPort  ActionType=else
  Out1 : Outport
  wires:
  In1/1 -> Out1/1

== system SF050A_MotTqTranlDampg/MotTqTranlDampg/MotTqTranlDampgPer1/CompDmpTrq/PhasePlaneSwitching/CopyRight2 ==

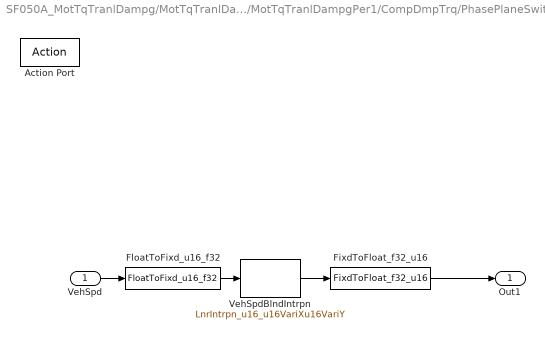
== system SF050A_MotTqTranlDampg/MotTqTranlDampg/MotTqTranlDampgPer1/CompDmpTrq/PhasePlaneSwitching/VehSpdBlnd_Intrpn ==
  VehSpd : Inport
  Action Port : ActionPort  ActionType=then
  FixdToFloat_f32_u16 : FixdToFloat/FixdToFloat_f32_u16  Param1=14
  FloatToFixd_u16_f32 : FloatToFixd/FloatToFixd_u16_f32  Param1=7
  VehSpdBlndIntrpn : LnrIntrpn/LnrIntrpn_u16_u16VariXu16VariY  XTbl=MotTqTranlDampgVehSpdBlndX  YTbl=MotTqTranlDampgVehSpdBlndY
      settings: AttributesFormatString=Lnr ( u16VariX , u16VariY )
  Out1 : Outport
  wires:
  VehSpd/1 -> FloatToFixd_u16_f32/1
  FloatToFixd_u16_f32/1 -> VehSpdBlndIntrpn/1
  VehSpdBlndIntrpn/1 -> FixdToFloat_f32_u16/1
  FixdToFloat_f32_u16/1 -> Out1/1
